simulink model "uebung2_population_Lukas"  (R2015a)
settings: Solver=ode45  StartTime=0.0  StopTime=500  RelTol=1e-3
settings Model: Creator=lustoppe  LastModifiedBy=lustoppe

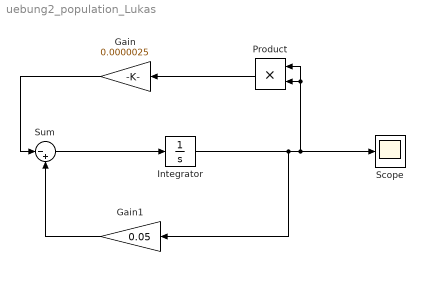
== system uebung2_population_Lukas ==
  Gain : Gain  Gain=0.0000025
  Gain1 : Gain  Gain=0.05
  Integrator : Integrator  InitialCondition=10000
  Product : Product
  Scope : Scope
      settings: TimeRange=60  YMin=0  YMax=100
  Sum : Sum  Inputs=|-+
  wires:
  Gain/1 -> Sum/1
  Gain1/1 -> Sum/2
  Sum/1 -> Integrator/1
  Product/1 -> Gain/1
  Integrator/1 -> Gain1/1, Scope/1, Product/1, Product/2
